simulink model "Full_Simulation"  (R2024a)
settings: Solver=FixedStepAuto  StartTime=0.0  StopTime=inf  FixedStep=0.001  MaxStep=0.001  RelTol=1e-3
model workspace: external: MATLAB File E:\Senior2\Hybrid\Project_Hybrid\Simulink_Bodies\Trial_5\Trial_5_DataFile.m (data not in the file)
values from neighbouring files (symbols this model uses):
  g = 9.81    [final_parameters.mat]
  J = 0.0024    [final_parameters.mat]
  Jr = 9.83e-05    [final_parameters.mat]
  k_sim = 2.5    [final_parameters.mat]
  Lr = 0.0638    [final_parameters.mat]
  mr = 0.018    [final_parameters.mat]
  smiData =     [final_parameters.mat]
undefined symbols (not defined in the file or in its folder): X, Y, Z
libraries: sm_lib x37, nesl_utility x10, fl_lib x5, simulink_extras x4, ee_lib x4, eeGeneralControl x2
(part 2 of 2)

== matlab function Full_Simulation/Subsystem/MATLAB Function2 ==
  data: tau input; pwm output; omega input
function pwm = torque_to_pwm(tau, omega)

% === Motor parameters (estimated) ===
Kt = (12/250)*60/(2*pi);       % Nm/A
Ke = Kt;       % V/(rad/s)
R  =  5.8466;        % Ohms
Vmax = 12;       % Supply voltage

% === Torque → Voltage ===
V = (tau / Kt) * R + Ke * omega;

% === Voltage → PWM ===
pwm = 255 * V / Vmax;

% === Saturation ===
pwm = max(min(pwm,180),-180);

end
